simulink model "lab1_simulink"  (R2022a)
settings: Solver=ode23t  StartTime=0.0  StopTime=0.05  MaxStep=1e-5  RelTol=1e-3
values from neighbouring files (symbols this model uses):
  C = 10e-6    (= 1e-05)    [lab1.m]
  Em = 24    [lab1.m]
  I_2_0 = 1    [lab1.m]
  L = 20e-3    (= 0.02)    [lab1.m]
  R1 = 12    [lab1.m]
  R2 = 15    [lab1.m]
  U_C_0 = 1    [lab1.m]
  w = 50*2*pi    (= 314.159265359)    [lab1.m]
libraries: fl_lib x7, nesl_utility x4, ee_lib x1
settings Model: Creator=81502  LastModifiedBy=81502

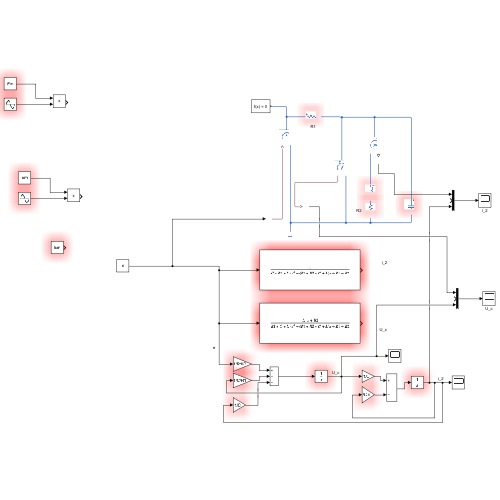
[thumbnail: Simulink's stored preview of the top-level diagram]
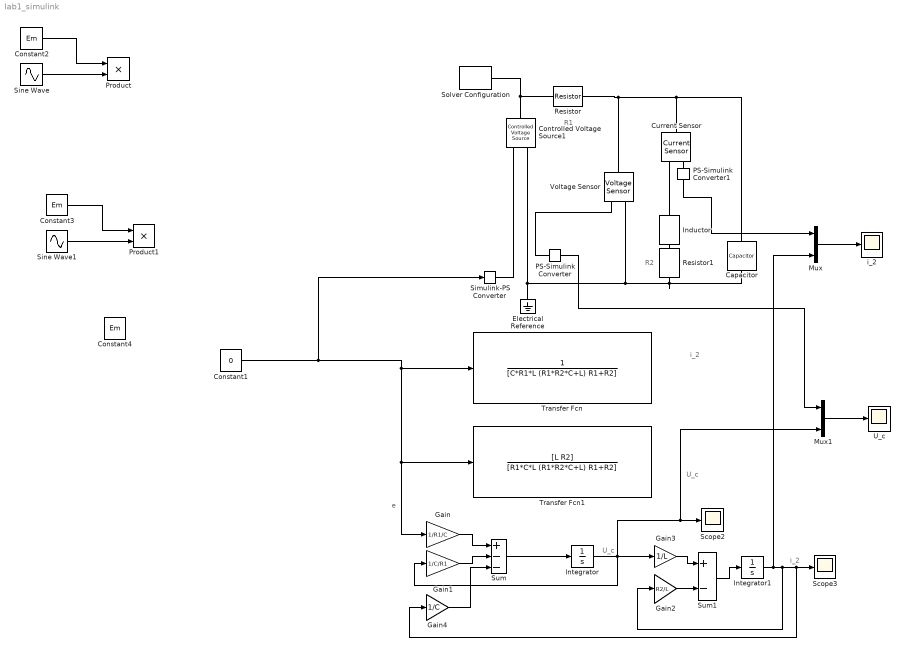
== system lab1_simulink ==
  note: e
  note: U_c
  note: i_2
  note: U_c
  note: i_2
  note: R2
  note: R1
  Capacitor : fl_lib/Electrical/Electrical Elements/Capacitor  c=C F  r=1e-6 Ohm  g=0 1/Ohm  i_specify=off  i_priority=None  i=0 A  i_nominal_specify=off  i_nominal_unit=A  i_nominal_value=1  v_specify=on  v_priority=High  v=U_C_0 V  v_nominal_specify=off  v_nominal_unit=V  v_nominal_value=1  vc_specify=off  vc_priority=High  vc=U_C_0 V  vc_nominal_specify=off  vc_nominal_unit=V  vc_nominal_value=1
      settings: SourceProductBaseCode=PW,SS,VE
  Constant1 : Constant  Value=0
  Constant2 : Constant  Value=Em
  Constant3 : Constant  Value=Em
  Constant4 : Constant  Value=Em
  Controlled Voltage Source1 : fl_lib/Electrical/Electrical Sources/Controlled Voltage Source
      settings: SourceProductBaseCode=PW,SS,VE
  Current Sensor : fl_lib/Electrical/Electrical Sensors/Current Sensor
      settings: SourceProductBaseCode=PW,SS,VE
  Electrical Reference : fl_lib/Electrical/Electrical Elements/Electrical Reference
      settings: SourceProductBaseCode=PW,SS,VE
  Gain : Gain  Gain=1/R1/C
  Gain1 : Gain  Gain=1/C/R1
  Gain2 : Gain  Gain=R2/L
  Gain3 : Gain  Gain=1/L
  Gain4 : Gain  Gain=1/C
  Inductor : ee_lib/Passive/Inductor  l=L H  enable_L_tol=0  L_tol=20  tol_distribution=1  nSigma=4  r=0 Ohm  g=1e-9 1/Ohm  enable_operating_limits=0  operating_limit_action=2  max_working_current=1 A  power_rating=1 W  enable_faults=0  fault_action=1  lambdaPercent=50  k_faulted=0.9999  turnsShort=0  openCct=0  groundShort=0  groundShortG=0 1/Ohm  tau_fault=1e-3 s  enable_temporal_fault=0  t_fault=1 s  enable_behavioral_fault=0  max_permissible_voltage=100 V  n_fail_on_voltage=1  max_permissible_current=1 A  t_fail_on_current=1 s  i_L_specify=on  i_L_priority=High  i_L=I_2_0 A  i_L_nominal_specify=off  i_L_nominal_unit=A  i_L_nominal_value=1
  Integrator : Integrator  InitialCondition=U_C_0
  Integrator1 : Integrator  InitialCondition=I_2_0
  Mux : Mux  Inputs=3
  Mux1 : Mux  Inputs=3
  PS-Simulink Converter : nesl_utility/PS-Simulink Converter  PhysicalDomain=network_engine_domain  SubClassName=ps_output  LeftPortType=input  RightPortType=output  PseudoPeriodic=off  Frequencies=[]  VectorFormat=inherit  Unit=inherit  AffineConversion=off
      settings: SourceProductBaseCode=SS,PW,VE
  PS-Simulink Converter1 : nesl_utility/PS-Simulink Converter  PhysicalDomain=network_engine_domain  SubClassName=ps_output  LeftPortType=input  RightPortType=output  PseudoPeriodic=off  Frequencies=[]  VectorFormat=inherit  Unit=inherit  AffineConversion=off
      settings: SourceProductBaseCode=SS,PW,VE
  Product : Product
  Product1 : Product
  Resistor : fl_lib/Electrical/Electrical Elements/Resistor  R=R1 Ohm  i_specify=off  i_priority=None  i=0 A  i_nominal_specify=off  i_nominal_unit=A  i_nominal_value=1  v_specify=off  v_priority=None  v=0 V  v_nominal_specify=off  v_nominal_unit=V  v_nominal_value=1
      settings: SourceProductBaseCode=PW,SS,VE
  Resistor1 : fl_lib/Electrical/Electrical Elements/Resistor  R=R2 Ohm  i_specify=off  i_priority=None  i=0 A  i_nominal_specify=off  i_nominal_unit=A  i_nominal_value=1  v_specify=off  v_priority=None  v=0 V  v_nominal_specify=off  v_nominal_unit=V  v_nominal_value=1
      settings: SourceProductBaseCode=PW,SS,VE
  Scope2 : Scope
  Scope3 : Scope
  Simulink-PS Converter : nesl_utility/Simulink-PS Converter  PhysicalDomain=network_engine_domain  SubClassName=ps_input  LeftPortType=input  RightPortType=output  PseudoPeriodic=off  Frequencies=[]  NoiseDistribution=none  NoiseParameters=[]  Unit=1  AffineConversion=off  FilteringAndDerivatives=provide  SimscapeFilterOrder=1  InputFilterTimeConstant=0.001  UdotUserProvided=0
      settings: SourceProductBaseCode=SS,PW,VE
  Sine Wave : Sin  Frequency=w  SampleTime=0
  Sine Wave1 : Sin  Frequency=w  SampleTime=0
  Solver Configuration : nesl_utility/Solver Configuration  PhysicalDomain=network_engine_domain  SubClassName=solver  LeftPortType=input  RightPortType=generic  Tones=[]  Harmonics=[]  SimulateNoise=off  Profile=off  UseLocalSampling=off  EnableSwitchedLinearOptims=on  FrequencyDomain=off  UseCCode=off  RelTol=0.001  AbsTol=0.001  MinStep=1e-09  ToWorkspace=off  RevertToSquareIcSolve=off  NumHomotopyIterations=100  PhasorMode=off  PhasorModeNumHarmonics=1  IndexReductionMethod=DerivativeReplacement  DoDC=off  ResidualTolerance=1e-09  UseLocalSolver=off  LocalSolverChoice=NE_BACKWARD_EULER_ADVANCER  LocalSolverSampleTime=0.001  DoFixedCost=off  MaxNonlinIter=3  MaxModeIter=2  ComputeImpulses=off  ImpulseIterations=2  LinearAlgebra=auto  LinearAlgebraNumThread=0  EquationFormulation=NE_TIME_EF  DelaysMemoryBudget=1024  AutomaticFiltering=on  FilteringTimeConstant=0.001  PartitionStorageMethod=AS_NEEDED  PartitionMemoryBudget=1024  PartitionMethod=ROBUST
      settings: SourceProductBaseCode=SS,PW,VE
  Sum : Sum  Inputs=+--
  Sum1 : Sum  Inputs=+-
  Transfer Fcn : TransferFcn  Denominator=[C*R1*L (R1*R2*C+L) R1+R2]
  Transfer Fcn1 : TransferFcn  Numerator=[L R2]  Denominator=[R1*C*L (R1*R2*C+L) R1+R2]
  U_c : Scope
  Voltage Sensor : fl_lib/Electrical/Electrical Sensors/Voltage Sensor
      settings: SourceProductBaseCode=PW,SS,VE
  i_2 : Scope
  wires:
  PS-Simulink Converter/1 -> Mux1/1
  Gain/1 -> Sum/1
  Gain1/1 -> Sum/2
  Sum/1 -> Integrator/1
  Integrator/1 -> Gain1/1, Mux1/3, Scope2/1, Gain3/1
  Constant1/1 -> Simulink-PS Converter/1, Gain/1, Transfer Fcn1/1, Transfer Fcn/1
  PS-Simulink Converter1/1 -> Mux/1
  Gain3/1 -> Sum1/1
  Sum1/1 -> Integrator1/1
  Gain2/1 -> Sum1/2
  Gain4/1 -> Sum/3
  Integrator1/1 -> Mux/3, Scope3/1, Gain4/1, Gain2/1
  Mux/1 -> i_2/1
  Mux1/1 -> U_c/1
  Sine Wave/1 -> Product/2
  Constant2/1 -> Product/1
  Constant3/1 -> Product1/1
  Sine Wave1/1 -> Product1/2
  connections:
  Controlled Voltage Source1/LConn1 -- Resistor/LConn1 -- Solver Configuration/RConn1
  Electrical Reference/LConn1 -- Capacitor/RConn1 -- Resistor1/RConn1 -- Voltage Sensor/RConn2 -- Controlled Voltage Source1/RConn2
  Voltage Sensor/LConn1 -- Resistor/RConn1 -- Capacitor/LConn1 -- Current Sensor/LConn1
  Simulink-PS Converter/RConn1 -- Controlled Voltage Source1/RConn1
  Voltage Sensor/RConn1 -- PS-Simulink Converter/LConn1
  Inductor/RConn1 -- Resistor1/LConn1
  Current Sensor/RConn2 -- Inductor/LConn1
  PS-Simulink Converter1/LConn1 -- Current Sensor/RConn1
